simulink model "balanceCAO"  (R2019b)
settings: Solver=VariableStepAuto  StartTime=0.0  StopTime=2  RelTol=1e-3
values from neighbouring files (symbols this model uses):
  B = 0.033125    [Lame_worspace.mat]    (also in Launcher.m = 0.928190886807; Parameters.mat = 0.441493924538; Poutre_diff.m = 0.441493924538; Workspace_lame.mat = 0.441493924538)
  f = 12.17    [Launcher.m]    (also in Parameters.mat; Poutre_diff.m; Workspace_lame.mat)
  L = 0.24    [Lame_worspace.mat]    (also in Launcher.m; Parameters.mat; Poutre_diff.m; Workspace_lame.mat)
undefined symbols (not defined in the file or in its folder): D, I, I0, Kamp, Kc, Ke, N, R, Req, to, Voffset
settings Model: Creator=lucas  LastModifiedBy=lucas

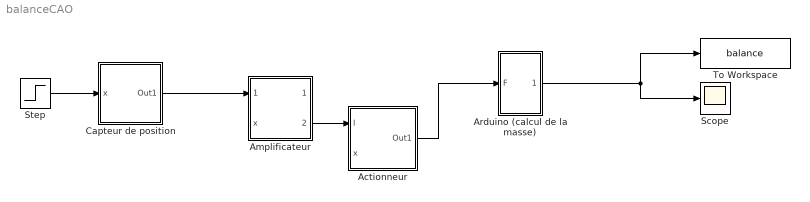
== system balanceCAO ==
  Actionneur : Subsystem  mask{B=B, D=D, N=N, f=f, J=I}
      mask prompts: B "Champ magnétique"; D "Diamètre"; N "Nombre de tour"; f "Coefficient de frottement"; J "Inertie"
  Amplificateur : Subsystem  mask{Voffset=Voffset, Kamp=Kamp, to=to, La=L, Req=Req, Ra=R, Ke=Ke, Kc=Kc, I0=I0}
      mask prompts: Voffset "Tension de offset"; Kamp "Gain de l'ampli audio"; to "Constante de temps de l'ampli audio"; La "Inductance de la bobine"; Req "Résistance équivalent de puissance"; Ra "Résistance de la bobine"; Ke "Constante contre-électromotrice"; Kc "Gain courant-tension"; I0 "Courant initial"
  Arduino (calcul de la masse) : Subsystem
  Capteur de position : Subsystem  mask{aO=0, dE=0, gA1=0, Vd1=0, fc=1, gA2=0, Vd2=0, eL=0.1, R1=0, R2=0, R3=0, R4=0}
      mask prompts: aO "Amplitude de l'onde carré de l'oscillateur"; dE "Distance entre les électrodes"; gA1 "Gain du 1er ampli"; Vd1 "Tension décalage 1er ampli"; fc "Fréquence de coupure du filtre"; gA2 "Gain du 2e ampli"; Vd2 "Tension décalage 2e ampli"; eL "Épaisseur de la lame"; R1 "Résistance 1"; R2 "Résistance 2"; R3 "Résistance 3"; R4 "Résistance 4"
  Scope : Scope
  Step : Step  SampleTime=0
  To Workspace : ToWorkspace  VariableName=balance  SaveFormat=Timeseries  SampleTime=-1
  wires:
  Actionneur/1(Out1) -> Arduino (calcul de la masse)/1(F)
  Arduino (calcul de la masse)/1(m (g)) -> To Workspace/1, Scope/1
  Amplificateur/2(actionneur) -> Actionneur/1(I)
  Capteur de position/1(Out1) -> Amplificateur/1(Vamp)
  Step/1 -> Capteur de position/1(x)

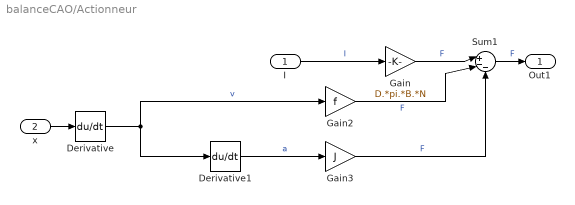
== system balanceCAO/Actionneur ==
  I : Inport
  x : Inport  Port=2
  Derivative : Derivative
  Derivative1 : Derivative
  Gain : Gain  Gain=D.*pi.*B.*N
  Gain2 : Gain  Gain=f
  Gain3 : Gain  Gain=J
  Sum1 : Sum  Inputs=|+--
  Out1 : Outport
  wires:
  I/1 -> Gain/1  "I"
  Gain/1 -> Sum1/1  "F"
  Derivative/1 -> Derivative1/1, Gain2/1  "v"
  x/1 -> Derivative/1
  Gain2/1 -> Sum1/2  "F"
  Derivative1/1 -> Gain3/1  "a"
  Gain3/1 -> Sum1/3  "F"
  Sum1/1 -> Out1/1  "F"

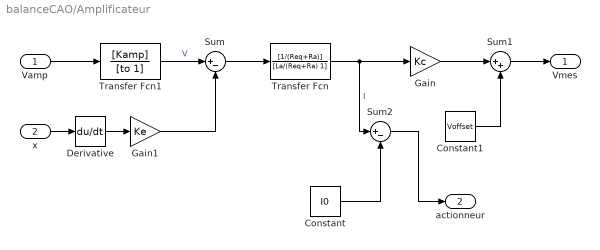
== system balanceCAO/Amplificateur ==
  Vamp : Inport
  x : Inport  Port=2
  Constant : Constant  Value=I0
  Constant1 : Constant  Value=Voffset
  Derivative : Derivative
  Gain : Gain  Gain=Kc
  Gain1 : Gain  Gain=Ke
  Sum : Sum  Inputs=|+-
  Sum1 : Sum  Inputs=|++
  Sum2 : Sum  Inputs=|+-
  Transfer Fcn : TransferFcn  Numerator=[1/(Req+Ra)]  Denominator=[La/(Req+Ra) 1]
  Transfer Fcn1 : TransferFcn  Numerator=[Kamp]  Denominator=[to 1]
  Vmes : Outport
  actionneur : Outport  Port=2
  wires:
  Sum1/1 -> Vmes/1
  Constant1/1 -> Sum1/2
  Transfer Fcn1/1 -> Sum/1  "V"
  Vamp/1 -> Transfer Fcn1/1
  x/1 -> Derivative/1
  Derivative/1 -> Gain1/1
  Gain1/1 -> Sum/2
  Sum/1 -> Transfer Fcn/1
  Transfer Fcn/1 -> Sum2/1, Gain/1  "I"
  Gain/1 -> Sum1/1
  Sum2/1 -> actionneur/1
  Constant/1 -> Sum2/2

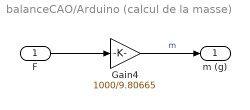
== system balanceCAO/Arduino (calcul de la masse) ==
  F : Inport
  Gain4 : Gain  Gain=1000/9.80665
  m (g) : Outport
  wires:
  Gain4/1 -> m (g)/1  "m"
  F/1 -> Gain4/1

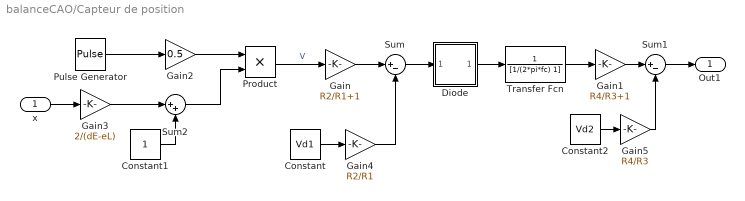
== system balanceCAO/Capteur de position ==
  x : Inport
  Constant : Constant  Value=Vd1
  Constant1 : Constant
  Constant2 : Constant  Value=Vd2
  Diode : Subsystem
  Gain : Gain  Gain=R2/R1+1
  Gain1 : Gain  Gain=R4/R3+1
  Gain2 : Gain  Gain=0.5
  Gain3 : Gain  Gain=2/(dE-eL)
  Gain4 : Gain  Gain=R2/R1
  Gain5 : Gain  Gain=R4/R3
  Product : Product
  Pulse Generator : DiscretePulseGenerator  PulseType=Time based  Amplitude=aO  Period=0.0000001  PulseWidth=50
  Sum : Sum  Inputs=|+-
  Sum1 : Sum  Inputs=|+-
  Sum2 : Sum  Inputs=|++
  Transfer Fcn : TransferFcn  Denominator=[1/(2*pi*fc) 1]
  Out1 : Outport
  wires:
  Pulse Generator/1 -> Gain2/1
  Gain2/1 -> Product/1
  Constant1/1 -> Sum2/2
  x/1 -> Gain3/1
  Gain3/1 -> Sum2/1
  Sum2/1 -> Product/2
  Product/1 -> Gain/1  "V"
  Gain/1 -> Sum/1
  Gain1/1 -> Sum1/1
  Sum/1 -> Diode/1(In1)
  Diode/1(Out1) -> Transfer Fcn/1
  Transfer Fcn/1 -> Gain1/1
  Sum1/1 -> Out1/1
  Constant/1 -> Gain4/1
  Gain4/1 -> Sum/2
  Constant2/1 -> Gain5/1
  Gain5/1 -> Sum1/2

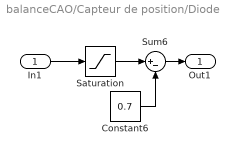
== system balanceCAO/Capteur de position/Diode ==
  In1 : Inport
  Constant6 : Constant  Value=0.7
  Saturation : Saturate  UpperLimit=inf  LowerLimit=0.7
  Sum6 : Sum  Inputs=|+-
  Out1 : Outport
  wires:
  Saturation/1 -> Sum6/1
  Constant6/1 -> Sum6/2
  Sum6/1 -> Out1/1
  In1/1 -> Saturation/1
